simulink model "untitled"  (R2015a)
settings: Solver=ode4  StartTime=0.0  StopTime=10.0  FixedStep=1e-3  RelTol=1e-3
libraries: fl_lib x12, nesl_utility x3
settings Model: Creator=Jesus  LastModifiedBy=Jesus

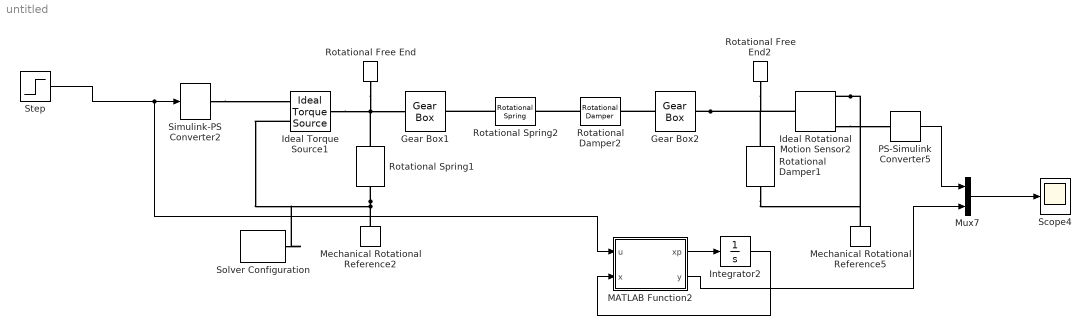
== system untitled ==
  Gear Box1 : fl_lib/Mechanical/Mechanisms/Gear Box  ratio=300/30  t_in_specify=off  t_in_priority=High  t_in=0 N*m  t_out_specify=off  t_out_priority=High  t_out=0 N*m
  Gear Box2 : fl_lib/Mechanical/Mechanisms/Gear Box  ratio=100/10  t_in_specify=off  t_in_priority=High  t_in=0 N*m  t_out_specify=off  t_out_priority=High  t_out=0 N*m
  Ideal Rotational Motion Sensor2 : fl_lib/Mechanical/Mechanical Sensors/Ideal Rotational Motion Sensor  offset=0 rad
  Ideal Torque Source1 : fl_lib/Mechanical/Mechanical Sources/Ideal Torque Source
  Integrator2 : Integrator  InitialCondition=[0;0]
  MATLAB Function2 : MATLAB Function  TreatAsAtomicUnit=on
  Mechanical Rotational Reference2 : fl_lib/Mechanical/Rotational Elements/Mechanical Rotational Reference
  Mechanical Rotational Reference5 : fl_lib/Mechanical/Rotational Elements/Mechanical Rotational Reference
  Mux7 : Mux  Inputs=2
  PS-Simulink Converter5 : nesl_utility/PS-Simulink Converter  PhysicalDomain=network_engine_domain  SubClassName=ps_output  LeftPortType=input  RightPortType=output  PseudoPeriodic=off  Frequencies=[]  Unit=1  AffineConversion=off
  Rotational Damper1 : fl_lib/Mechanical/Rotational Elements/Rotational Damper  D=200 N*m/(rad/s)  w_specify=off  w_priority=High  w=0 rad/s  t_specify=off  t_priority=High  t=0 N*m
  Rotational Damper2 : fl_lib/Mechanical/Rotational Elements/Rotational Damper  D=3 N*m/(rad/s)  w_specify=off  w_priority=High  w=0 rad/s  t_specify=off  t_priority=High  t=0 N*m
  Rotational Free End : fl_lib/Mechanical/Rotational Elements/Rotational Free End  w_specify=on  w_priority=High  w=0 rad/s
  Rotational Free End2 : fl_lib/Mechanical/Rotational Elements/Rotational Free End  w_specify=on  w_priority=High  w=0 rad/s
  Rotational Spring1 : fl_lib/Mechanical/Rotational Elements/Rotational Spring  spr_rate=1/10 N*m/rad  w_specify=off  w_priority=High  w=0 rad/s  t_specify=off  t_priority=High  t=0 N*m  phi_specify=off  phi_priority=High  phi=0 rad
  Rotational Spring2 : fl_lib/Mechanical/Rotational Elements/Rotational Spring  spr_rate=2 N*m/rad  w_specify=off  w_priority=High  w=0 rad/s  t_specify=off  t_priority=High  t=0 N*m  phi_specify=off  phi_priority=High  phi=0 rad
  Scope4 : Scope
      settings: YMin=2.27  YMax=2.48  SaveName=ScopeData4
  Simulink-PS Converter2 : nesl_utility/Simulink-PS Converter  PhysicalDomain=network_engine_domain  SubClassName=ps_input  LeftPortType=input  RightPortType=output  PseudoPeriodic=off  Frequencies=[]  NoiseDistribution=none  NoiseParameters=[]  Unit=1  AffineConversion=off  InputFiltering=off  SimscapeFilterOrder=1  InputFilterTimeConstant=0.001  UdotUserProvided=1
  Solver Configuration : nesl_utility/Solver Configuration  PhysicalDomain=network_engine_domain  SubClassName=solver  LeftPortType=input  RightPortType=generic  Accelerate=off  Tones=[]  Harmonics=[]  SimulateNoise=off  Profile=off  UseLocalSampling=off  EnableSwitchedLinearOptims=on  FrequencyDomain=off  UseCCode=off  RelTol=0.001  AbsTol=1e-06  MinStep=1e-09  ToWorkspace=off  RevertToSquareIcSolve=off  NumHomotopyIterations=100  DoDC=off  ResidualTolerance=1e-09  UseLocalSolver=on  LocalSolverChoice=NE_BACKWARD_EULER_ADVANCER  LocalSolverSampleTime=0.001  DoFixedCost=on  MaxNonlinIter=3  MaxModeIter=2  LinearAlgebra=Sparse  DelaysMemoryBudget=1024  AutomaticFiltering=on  FilteringTimeConstant=0.001
  Step : Step  SampleTime=0
  wires:
  MATLAB Function2/1(xp) -> Integrator2/1
  Integrator2/1 -> MATLAB Function2/2(x)
  PS-Simulink Converter5/1 -> Mux7/1
  Mux7/1 -> Scope4/1
  MATLAB Function2/2(y) -> Mux7/2
  Step/1 -> MATLAB Function2/1(u), Simulink-PS Converter2/1
  connections:
  Ideal Torque Source1/LConn1 -- Rotational Spring1/LConn1 -- Rotational Free End/LConn1 -- Gear Box1/LConn1
  Rotational Spring1/RConn1 -- Ideal Torque Source1/RConn2 -- Solver Configuration/RConn1 -- Mechanical Rotational Reference2/LConn1
  Gear Box2/RConn1 -- Rotational Damper1/LConn1 -- Rotational Free End2/LConn1 -- Ideal Rotational Motion Sensor2/LConn1
  Ideal Rotational Motion Sensor2/RConn1 -- Rotational Damper1/RConn1 -- Mechanical Rotational Reference5/LConn1
  Gear Box2/LConn1 -- Rotational Damper2/RConn1
  Ideal Rotational Motion Sensor2/RConn3 -- PS-Simulink Converter5/LConn1
  Rotational Damper2/LConn1 -- Rotational Spring2/RConn1
  Simulink-PS Converter2/RConn1 -- Ideal Torque Source1/RConn1
  Rotational Spring2/LConn1 -- Gear Box1/RConn1

== matlab function untitled/MATLAB Function2 ==
  data: xp output; u input; y output; x input
function [xp,y] = fcn(u,x)
%#codegen
A=[-25/18 0;-5/6 0];
B=[25/18 5/6]';
C=[0 1/10];
xp=A*x+B*u;
y = C*x;
